simulink model "BobbyCar_mod"  (Simulink 7.9)
settings: Solver=ode45  StartTime=0.0  StopTime=10.0  RelTol=1e-3
values from neighbouring files (symbols this model uses):
  A = 0.4    [BobbyCar_dat.m]
  cw = 0.6    [BobbyCar_dat.m]
  F = 80    [BobbyCar_dat.m]
  FR = 10    [BobbyCar_dat.m]
  m = 35    [BobbyCar_dat.m]
  v_50 = 50*1000/3600    (= 13.8888888889)    [BobbyCar_dat.m]
libraries: simulink x2
settings Model: Creator=Andreas  LastModifiedBy=Andreas

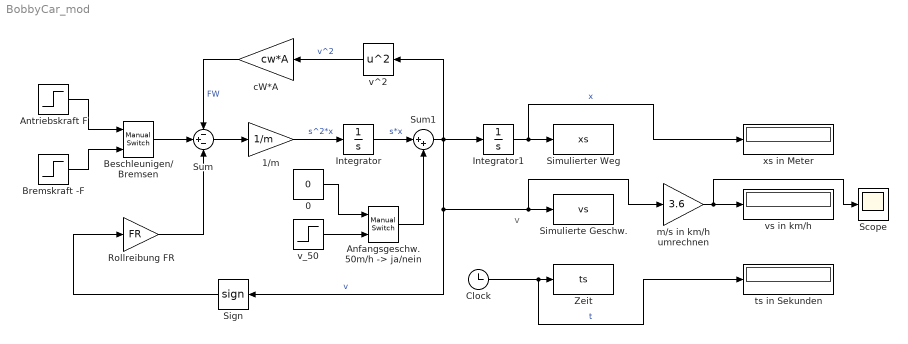
== system BobbyCar_mod ==
  note: v
  0 : Constant  Value=0
  1/m : Gain  Gain=1/m
  "Anfangsgeschw. 50m/h -> ja/nein" : simulink/Signal Routing/Manual Switch  sw=1  action=0  varsize=off
  Antriebskraft F : Step  Time=0  After=F  SampleTime=0
  Beschleunigen/ Bremsen : simulink/Signal Routing/Manual Switch  sw=1  action=0  varsize=off
  Bremskraft -F : Step  Time=0  After=-F  SampleTime=0
  Clock : Clock
  Integrator : Integrator
  Integrator1 : Integrator
  Rollreibung FR : Gain  Gain=FR
  Scope : Scope
      settings: TimeRange=30  YMin=0  YMax=110
  Sign : Signum
  Simulierte Geschw. : ToWorkspace  VariableName=vs  SampleTime=-1
  Simulierter Weg : ToWorkspace  VariableName=xs  SampleTime=-1
  Sum : Sum  Inputs=-+-
  Sum1 : Sum  Inputs=|++
  Zeit : ToWorkspace  VariableName=ts  SampleTime=-1
  cW*A : Gain  Gain=cw*A
  m/s in km/h umrechnen : Gain  Gain=3.6
  ts in Sekunden : Display
  v^2 : Math  Operator=square  SaturateOnIntegerOverflow=on
  v_50 : Step  Time=0  After=v_50  SampleTime=0
  vs in km/h : Display
  xs in Meter : Display
  wires:
  Sum/1 -> 1/m/1
  1/m/1 -> Integrator/1  "s^2*x"
  Integrator1/1 -> Simulierter Weg/1, xs in Meter/1  "x"
  v^2/1 -> cW*A/1  "v^2"
  cW*A/1 -> Sum/1  "FW"
  Clock/1 -> Zeit/1, ts in Sekunden/1  "t"
  Integrator/1 -> Sum1/1  "s*x"
  Sum1/1 -> Integrator1/1, Simulierte Geschw./1, m/s in km/h umrechnen/1, Sign/1, v^2/1  "v"
  "Anfangsgeschw. 50m/h -> ja/nein"/1 -> Sum1/2
  v_50/1 -> "Anfangsgeschw. 50m/h -> ja/nein"/2
  Sign/1 -> Rollreibung FR/1
  Rollreibung FR/1 -> Sum/3
  Beschleunigen/ Bremsen/1 -> Sum/2
  Antriebskraft F/1 -> Beschleunigen/ Bremsen/1
  Bremskraft -F/1 -> Beschleunigen/ Bremsen/2
  m/s in km/h umrechnen/1 -> vs in km/h/1, Scope/1
  0/1 -> "Anfangsgeschw. 50m/h -> ja/nein"/1
